simulink model "que1"  (R2020b)
settings: Solver=VariableStepAuto  StartTime=0.0  StopTime=10.0  RelTol=1e-3
settings Model: Creator=ANUJA  LastModifiedBy=ANUJA

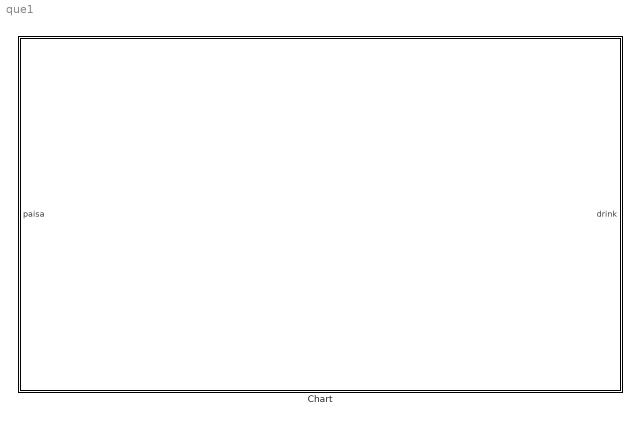
== system que1 ==
  Chart : Stateflow chart  TreatAsAtomicUnit=on

== stateflow chart que1/Chart ==
  state got_0
  state got_nickel
  state got_dime
  (default) -> got_0
  got_0 -> got_nickel [order 1] : [paisa==1]{drink=0}
  got_nickel -> got_0 [order 2] : [paisa==2]{drink=1}
  got_dime -> got_0 [order 1] : [paisa==1]{drink=1}
  got_0 -> got_dime [order 2] : [paisa==2]{drink=0}
  got_nickel -> got_dime [order 1] : [paisa==1]{drink=0}
  got_dime -> got_nickel [order 2] : [paisa==2]{drink=1}
  data: paisa input; drink output
